simulink model "P3"  (R2020b)
settings: Solver=VariableStepAuto  StartTime=0.0  StopTime=10.0  RelTol=1e-3
settings Model: Creator=ASUS  LastModifiedBy=ASUS

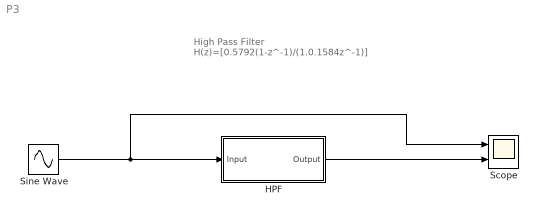
== system P3 ==
  note: High Pass Filter
      | H(z)=[0.5792(1-z^-1)/(1.0.1584z^-1)]
  HPF : Subsystem
  Scope : Scope  NumInputPorts=2
  Sine Wave : Sin  SampleTime=0
  wires:
  HPF/1(Output) -> Scope/2
  Sine Wave/1 -> Scope/1, HPF/1(Input)

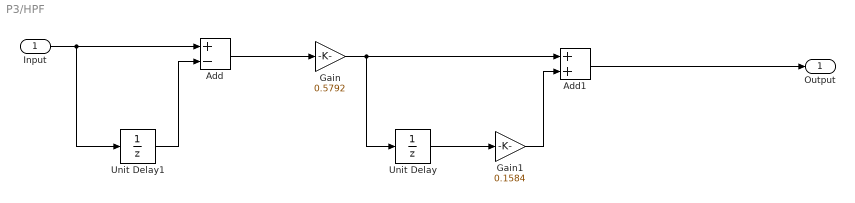
== system P3/HPF ==
  Input : Inport
  Add : Sum  Inputs=+-
  Add1 : Sum
  Gain : Gain  Gain=0.5792
  Gain1 : Gain  Gain=0.1584
  Unit Delay : UnitDelay  SampleTime=-1  HasFrameUpgradeWarning=on
  Unit Delay1 : UnitDelay  SampleTime=-1  HasFrameUpgradeWarning=on
  Output : Outport
  wires:
  Unit Delay/1 -> Gain1/1
  Gain/1 -> Unit Delay/1, Add1/1
  Add1/1 -> Output/1
  Gain1/1 -> Add1/2
  Add/1 -> Gain/1
  Unit Delay1/1 -> Add/2
  Input/1 -> Unit Delay1/1, Add/1
